simulink model "psis_pwm"  (R2020b)
settings: Solver=ode45  StartTime=0.0  StopTime=0.05  RelTol=1e-6  EnableMultiTasking=on
values from neighbouring files (symbols this model uses):
  f = 50 / 2    (= 25)    [task1.m]
  Ls = 0.087    [task1.m]
  Rs = 0.5    [task1.m]
  Ts = 0.002    [task1.m]
  Udc = 600    [task1.m]
  uftopp = 325 / 2    (= 162.5)    [task1.m]
settings Model: Creator=ielolof  LastModifiedBy=axelfroborg
settings DataIOCC: LimitDataPoints=on  SaveFormat=Array  SignalLoggingSaveFormat=ModelDataLogs  ReturnWorkspaceOutputs=off  SignalLoggingName=sigsOut
settings OptimizationCC: ExpressionDepthLimit=2147483647  InitFltsAndDblsToZero=on  LifeSpan=inf
settings DebuggingCC: SaveWithParameterizedLinksMsg=none  UnderspecifiedInitializationDetection=Classic  MergeDetectMultiDrivingBlocksExec=none  SignalResolutionControl=TryResolveAllWithWarning  MultiTaskDSMMsg=warning  MultiTaskCondExecSysMsg=none  FcnCallInpInsideContextMsg=warning  StateNameClashWarn=warning  SFUnexpectedBacktrackingDiag=warning  SFNoUnconditionalDefaultTransitionDiag=warning  SFExecutionAtInitializationDiag=none  ArithmeticOperatorsInVariantConditions=warning
settings HardwareCC: ProdBitPerPointer=32  ProdBitPerSizeT=32  ProdBitPerPtrDiffT=32  ProdLargestAtomicFloat=None  ProdIntDivRoundTo=Undefined  ProdEndianess=Unspecified  ProdWordSize=32  ProdHWDeviceType=32-bit Generic  TargetUnknown=on
settings ModelReferenceCC: PropagateSignalLabelsOutOfModel=off
settings SFSimCC: SimUseLocalCustomCode=off  CustomCodeUndefinedFunction=UseInterfaceOnly
settings RTWCC: RTWUseLocalCustomCode=off
settings CodeAppCC: StateflowObjectComments=on
settings GRTTargetCC: TargetLangStandard=C89/C90 (ANSI)  ModelReferenceCompliant=off  CompOptLevelCompliant=off  CombineOutputUpdateFcns=off  MatFileLogging=off  GRTInterface=on
settings ConfigComp: CovMetricSettings=dw  CovSaveCumulativeToWorkspaceVar=on  CovSaveSingleToWorkspaceVar=on  CovExternalEMLEnable=off  CovSFcnEnable=off

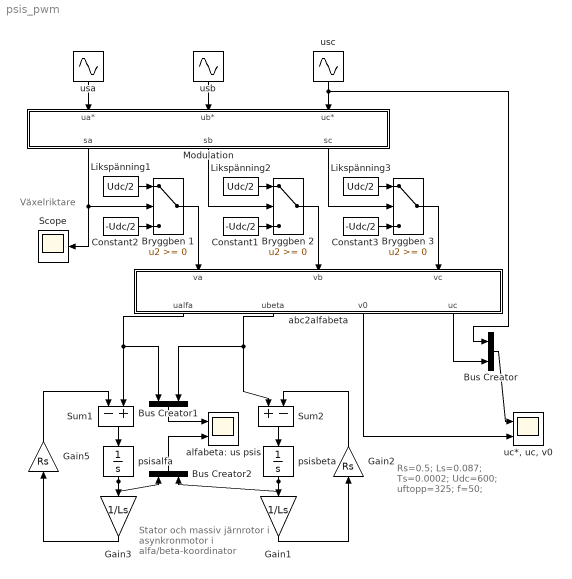
== system psis_pwm ==
  note: Rs=0.5;
      | Ls=0.087;
      | Ts=0.0002;
      | Udc=600;
      | uftopp=325;
      | f=50;
  note: Stator och massiv järnrotor
      | i asynkronmotor
      | i alfa/beta-koordinator
  note: Växelriktare
  Bryggben 1 : Switch  SaturateOnIntegerOverflow=on  InputSameDT=on
  Bryggben 2 : Switch  SaturateOnIntegerOverflow=on  InputSameDT=on
  Bryggben 3 : Switch  SaturateOnIntegerOverflow=on  InputSameDT=on
  Bus Creator : BusCreator  Inputs=2
  Bus Creator1 : BusCreator  Inputs=2
  Bus Creator2 : BusCreator  Inputs=2
  Constant1 : Constant  Value=-Udc/2
  Constant2 : Constant  Value=-Udc/2
  Constant3 : Constant  Value=-Udc/2
  Gain1 : Gain  Gain=1/Ls  SaturateOnIntegerOverflow=on  OutDataTypeStr=Inherit: Same as input  ParamDataTypeStr=Inherit: Same as input
  Gain2 : Gain  Gain=Rs  SaturateOnIntegerOverflow=on  OutDataTypeStr=Inherit: Same as input  ParamDataTypeStr=Inherit: Same as input
  Gain3 : Gain  Gain=1/Ls  SaturateOnIntegerOverflow=on  OutDataTypeStr=Inherit: Same as input  ParamDataTypeStr=Inherit: Same as input
  Gain5 : Gain  Gain=Rs  SaturateOnIntegerOverflow=on  OutDataTypeStr=Inherit: Same as input  ParamDataTypeStr=Inherit: Same as input
  Likspänning1 : Constant  Value=Udc/2
  Likspänning2 : Constant  Value=Udc/2
  Likspänning3 : Constant  Value=Udc/2
  Modulation : Subsystem
  Scope : Scope
  Sum1 : Sum  Inputs=-+  SaturateOnIntegerOverflow=on
  Sum2 : Sum  Inputs=+-  SaturateOnIntegerOverflow=on
  abc2alfabeta : Subsystem
  alfabeta: us psis : Scope  NumInputPorts=2
  psisalfa : Integrator  InitialCondition=-1.24
  psisbeta : Integrator
  "uc*, uc, v0" : Scope  NumInputPorts=2
  usa : Sin  Amplitude=uftopp  Frequency=2*pi*f  SampleTime=0
  usb : Sin  Amplitude=uftopp  Frequency=2*pi*f  Phase=-2*pi/3  SampleTime=0
  usc : Sin  Amplitude=uftopp  Frequency=2*pi*f  Phase=-4*pi/3  SampleTime=0
  wires:
  Sum1/1 -> psisalfa/1
  psisalfa/1 -> Gain3/1, Bus Creator2/1
  Gain3/1 -> Gain5/1
  Gain5/1 -> Sum1/1
  Constant2/1 -> Bryggben 1/3
  Modulation/1(sa) -> Bryggben 1/2, Scope/1
  Likspänning1/1 -> Bryggben 1/1
  usa/1 -> Modulation/1(ua*)
  usb/1 -> Modulation/2(ub*)
  usc/1 -> Modulation/3(uc*), Bus Creator/1
  Constant1/1 -> Bryggben 2/3
  Modulation/2(sb) -> Bryggben 2/2
  Likspänning2/1 -> Bryggben 2/1
  Constant3/1 -> Bryggben 3/3
  Modulation/3(sc) -> Bryggben 3/2
  Likspänning3/1 -> Bryggben 3/1
  abc2alfabeta/1(ualfa) -> Sum1/2, Bus Creator1/1
  Sum2/1 -> psisbeta/1
  psisbeta/1 -> Gain1/1, Bus Creator2/2
  Gain1/1 -> Gain2/1
  Gain2/1 -> Sum2/2
  abc2alfabeta/2(ubeta) -> Sum2/1, Bus Creator1/2
  Bryggben 1/1 -> abc2alfabeta/1(va)
  Bryggben 2/1 -> abc2alfabeta/2(vb)
  Bryggben 3/1 -> abc2alfabeta/3(vc)
  Bus Creator1/1 -> alfabeta: us psis/1
  Bus Creator2/1 -> alfabeta: us psis/2
  Bus Creator/1 -> "uc*, uc, v0"/1
  abc2alfabeta/3(v0) -> "uc*, uc, v0"/2
  abc2alfabeta/4(uc) -> Bus Creator/2

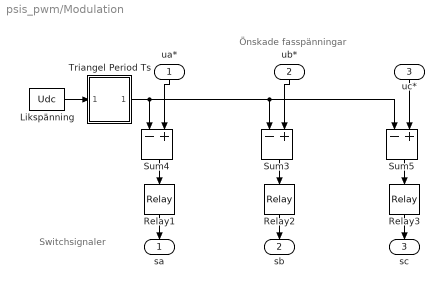
== system psis_pwm/Modulation ==
  note: Switchsignaler
  note: Önskade fasspänningar
  ua* : Inport
  ub* : Inport  Port=2
  uc* : Inport  Port=3
  Likspänning : Constant  Value=Udc
  Relay1 : Relay  OnOutputValue=1.01  OffOutputValue=-0.001
  Relay2 : Relay  OnOutputValue=1.01  OffOutputValue=-0.01
  Relay3 : Relay  OnOutputValue=1.01  OffOutputValue=-0.01
  Sum3 : Sum  Inputs=-+  InputSameDT=on  SaturateOnIntegerOverflow=on  OutDataTypeStr=Inherit: Same as first input
  Sum4 : Sum  Inputs=-+  InputSameDT=on  SaturateOnIntegerOverflow=on  OutDataTypeStr=Inherit: Same as first input
  Sum5 : Sum  Inputs=-+  InputSameDT=on  SaturateOnIntegerOverflow=on  OutDataTypeStr=Inherit: Same as first input
  Triangel Period Ts : Subsystem
  sa : Outport  VectorParamsAs1DForOutWhenUnconnected=off
  sb : Outport  Port=2  VectorParamsAs1DForOutWhenUnconnected=off
  sc : Outport  Port=3  VectorParamsAs1DForOutWhenUnconnected=off
  wires:
  Sum4/1 -> Relay1/1
  Triangel Period Ts/1(um) -> Sum4/1, Sum3/1, Sum5/1
  Likspänning/1 -> Triangel Period Ts/1(Udc)
  Sum3/1 -> Relay2/1
  Sum5/1 -> Relay3/1
  ub*/1 -> Sum3/2
  ua*/1 -> Sum4/2
  uc*/1 -> Sum5/2
  Relay1/1 -> sa/1
  Relay2/1 -> sb/1
  Relay3/1 -> sc/1

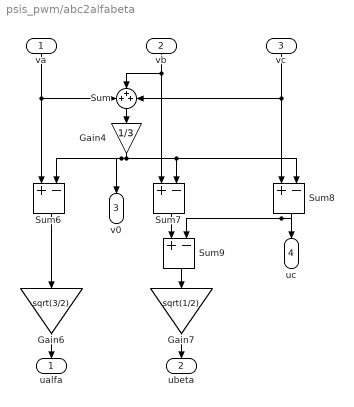
== system psis_pwm/abc2alfabeta ==
  va : Inport
  vb : Inport  Port=2
  vc : Inport  Port=3
  Gain4 : Gain  Gain=1/3  SaturateOnIntegerOverflow=on  OutDataTypeStr=Inherit: Same as input  ParamDataTypeStr=Inherit: Same as input
  Gain6 : Gain  Gain=sqrt(3/2)  SaturateOnIntegerOverflow=on  OutDataTypeStr=Inherit: Same as input  ParamDataTypeStr=Inherit: Same as input
  Gain7 : Gain  Gain=sqrt(1/2)  SaturateOnIntegerOverflow=on  OutDataTypeStr=Inherit: Same as input  ParamDataTypeStr=Inherit: Same as input
  Sum : Sum  Inputs=+++
  Sum{6..9} (4 alike) : Sum  Inputs=+-  InputSameDT=on  SaturateOnIntegerOverflow=on  OutDataTypeStr=Inherit: Same as first input
  ualfa : Outport  VectorParamsAs1DForOutWhenUnconnected=off
  ubeta : Outport  Port=2  VectorParamsAs1DForOutWhenUnconnected=off
  v0 : Outport  Port=3  VectorParamsAs1DForOutWhenUnconnected=off
  uc : Outport  Port=4  VectorParamsAs1DForOutWhenUnconnected=off
  wires:
  va/1 -> Sum6/1, Sum/1
  vc/1 -> Sum8/1, Sum/3
  vb/1 -> Sum7/1, Sum/2
  Sum/1 -> Gain4/1
  Gain4/1 -> Sum7/2, Sum8/2, Sum6/2, v0/1
  Sum6/1 -> Gain6/1
  Sum9/1 -> Gain7/1
  Sum7/1 -> Sum9/1
  Sum8/1 -> Sum9/2, uc/1
  Gain6/1 -> ualfa/1
  Gain7/1 -> ubeta/1

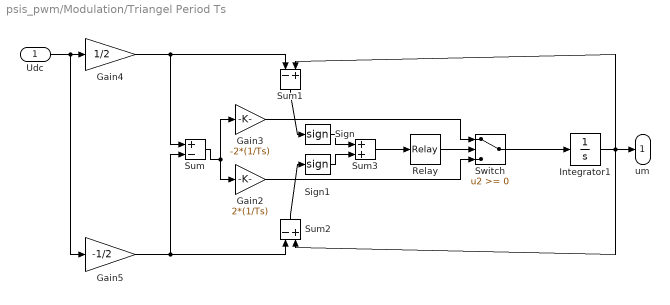
== system psis_pwm/Modulation/Triangel Period Ts ==
  Udc : Inport
  Gain2 : Gain  Gain=2*(1/Ts)  SaturateOnIntegerOverflow=on  OutDataTypeStr=Inherit: Same as input  ParamDataTypeStr=Inherit: Same as input
  Gain3 : Gain  Gain=-2*(1/Ts)  SaturateOnIntegerOverflow=on  OutDataTypeStr=Inherit: Same as input  ParamDataTypeStr=Inherit: Same as input
  Gain4 : Gain  Gain=1/2  SaturateOnIntegerOverflow=on  OutDataTypeStr=Inherit: Same as input  ParamDataTypeStr=Inherit: Same as input
  Gain5 : Gain  Gain=-1/2  SaturateOnIntegerOverflow=on  OutDataTypeStr=Inherit: Same as input  ParamDataTypeStr=Inherit: Same as input
  Integrator1 : Integrator
  Relay : Relay  OnSwitchValue=1  OffSwitchValue=-1  OffOutputValue=-1
  Sign : Signum
  Sign1 : Signum
  Sum : Sum  Inputs=+-  InputSameDT=on  SaturateOnIntegerOverflow=on  OutDataTypeStr=Inherit: Same as first input
  Sum1 : Sum  Inputs=-+  InputSameDT=on  SaturateOnIntegerOverflow=on  OutDataTypeStr=Inherit: Same as first input
  Sum2 : Sum  Inputs=-+  InputSameDT=on  SaturateOnIntegerOverflow=on  OutDataTypeStr=Inherit: Same as first input
  Sum3 : Sum  InputSameDT=on  SaturateOnIntegerOverflow=on  OutDataTypeStr=Inherit: Same as first input
  Switch : Switch  SaturateOnIntegerOverflow=on  InputSameDT=on
  um : Outport  VectorParamsAs1DForOutWhenUnconnected=off
  wires:
  Switch/1 -> Integrator1/1
  Gain3/1 -> Switch/1
  Gain2/1 -> Switch/3
  Integrator1/1 -> Sum1/2, Sum2/2, um/1
  Sum1/1 -> Sign/1
  Sum2/1 -> Sign1/1
  Sign/1 -> Sum3/1
  Sign1/1 -> Sum3/2
  Sum3/1 -> Relay/1
  Relay/1 -> Switch/2
  Sum/1 -> Gain3/1, Gain2/1
  Udc/1 -> Gain5/1, Gain4/1
  Gain5/1 -> Sum/2, Sum2/1
  Gain4/1 -> Sum/1, Sum1/1
